simulink model "wind_turbine_2021"  (R2024a)
settings: Solver=VariableStepAuto  StartTime=0.0  StopTime=20.0  RelTol=1e-3
values from neighbouring files (symbols this model uses):
  a1 = 0.4    [parameter_definition.m]
  a2 = 0.25    [parameter_definition.m]
  Cp_coef = coeffvalues(surf_fit)    [wind_turbine_sim.m]
  Ct_coef = coeffvalues(surf_fit)    [wind_turbine_sim.m]
  Kv = sqrt(2 * Tv * (1 - a2^2) / (a1^2/a2 - a2 + 1 - a1^2))    [parameter_definition.m]
  Noise_power = 1    [parameter_definition.m]
  Noise_Ts = 0.001    [parameter_definition.m]
  R = 125.88 / 2    (= 62.94)    [surface_fitting.m]
  Tv = Lm / Vm    (= 25)    [parameter_definition.m]
  Vm = 6    [parameter_definition.m]
undefined symbols (not defined in the file or in its folder): Nb, rho
libraries: simulink x1
settings Model: Creator=User  LastModifiedBy=ml4
settings OptimizationCC: ReuseModelBlockBuffer=off
settings RTWCC: GPUComputeCapability=3.5

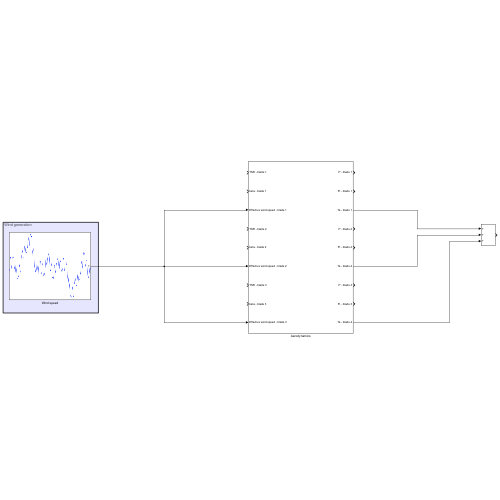
[thumbnail: Simulink's stored preview of the top-level diagram]
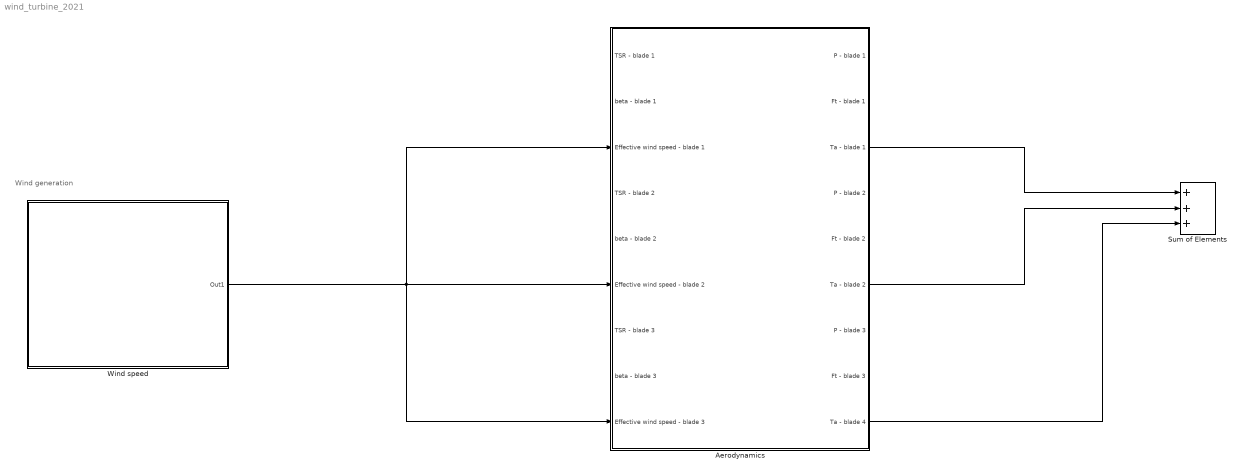
== system wind_turbine_2021 ==
  note: Wind generation
  Aerodynamics : Subsystem
  Sum of Elements : Sum  Inputs=+++
  Wind speed : Subsystem
      mask Display: image('./images/The-profile-of-the-wind-speed-versus-time.png');
  wires:
  Wind speed/1(Out1) -> Aerodynamics/3(Effective wind speed - blade 1), Aerodynamics/6(Effective wind speed - blade 2), Aerodynamics/9(Effective wind speed - blade 3)
  Aerodynamics/3(Ta - blade 1) -> Sum of Elements/1
  Aerodynamics/6(Ta - blade 2) -> Sum of Elements/2
  Aerodynamics/9(Ta - blade 4) -> Sum of Elements/3

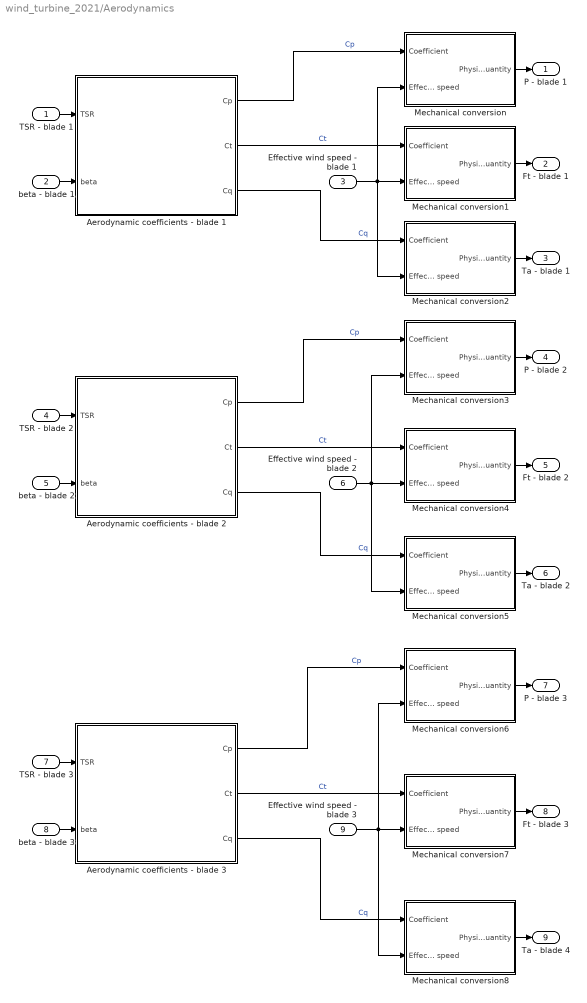
== system wind_turbine_2021/Aerodynamics ==
  TSR - blade 1 : Inport
  beta - blade 1 : Inport  Port=2
  Effective wind speed - blade 1 : Inport  Port=3
  TSR - blade 2 : Inport  Port=4
  beta - blade 2 : Inport  Port=5
  Effective wind speed - blade 2 : Inport  Port=6
  TSR - blade 3 : Inport  Port=7
  beta - blade 3 : Inport  Port=8
  Effective wind speed - blade 3 : Inport  Port=9
  Aerodynamic coefficients - blade 1 : Subsystem
      mask Display: image('C:\Users\User\Desktop\Project_repos\Controlab\Controlab\controlab\physical_models\2023\wind_turbine\images\Surface_fit.png'); % Use "Edit Image" on toolstrip to change.
  Aerodynamic coefficients - blade 2 : Subsystem
      mask Display: image('C:\Users\User\Desktop\Project_repos\Controlab\Controlab\controlab\physical_models\2023\wind_turbine\images\Surface_fit.png'); % Use "Edit Image" on toolstrip to change.
  Aerodynamic coefficients - blade 3 : Subsystem
      mask Display: image('C:\Users\User\Desktop\Project_repos\Controlab\Controlab\controlab\physical_models\2023\wind_turbine\images\Surface_fit.png'); % Use "Edit Image" on toolstrip to change.
  Mechanical conversion : Subsystem
  Mechanical conversion1 : Subsystem
  Mechanical conversion2 : Subsystem
  Mechanical conversion3 : Subsystem
  Mechanical conversion4 : Subsystem
  Mechanical conversion5 : Subsystem
  Mechanical conversion6 : Subsystem
  Mechanical conversion7 : Subsystem
  Mechanical conversion8 : Subsystem
  P - blade 1 : Outport
  Ft - blade 1 : Outport  Port=2
  Ta - blade 1 : Outport  Port=3
  P - blade 2 : Outport  Port=4
  Ft - blade 2 : Outport  Port=5
  Ta - blade 2 : Outport  Port=6
  P - blade 3 : Outport  Port=7
  Ft - blade 3 : Outport  Port=8
  Ta - blade 4 : Outport  Port=9
  wires:
  Aerodynamic coefficients - blade 1/1(Cp) -> Mechanical conversion/1(Coefficient)  "Cp"
  Aerodynamic coefficients - blade 3/3(Cq) -> Mechanical conversion8/1(Coefficient)  "Cq"
  Aerodynamic coefficients - blade 3/1(Cp) -> Mechanical conversion6/1(Coefficient)  "Cp"
  Aerodynamic coefficients - blade 3/2(Ct) -> Mechanical conversion7/1(Coefficient)  "Ct"
  beta - blade 1/1 -> Aerodynamic coefficients - blade 1/2(beta)
  Mechanical conversion5/1(Physical quantity) -> Ta - blade 2/1
  Aerodynamic coefficients - blade 2/3(Cq) -> Mechanical conversion5/1(Coefficient)  "Cq"
  Aerodynamic coefficients - blade 2/2(Ct) -> Mechanical conversion4/1(Coefficient)  "Ct"
  beta - blade 3/1 -> Aerodynamic coefficients - blade 3/2(beta)
  Aerodynamic coefficients - blade 2/1(Cp) -> Mechanical conversion3/1(Coefficient)  "Cp"
  Effective wind speed - blade 1/1 -> Mechanical conversion/2(Effective wind speed), Mechanical conversion1/2(Effective wind speed), Mechanical conversion2/2(Effective wind speed)
  Aerodynamic coefficients - blade 1/2(Ct) -> Mechanical conversion1/1(Coefficient)  "Ct"
  Aerodynamic coefficients - blade 1/3(Cq) -> Mechanical conversion2/1(Coefficient)  "Cq"
  TSR - blade 2/1 -> Aerodynamic coefficients - blade 2/1(TSR)
  Mechanical conversion6/1(Physical quantity) -> P - blade 3/1
  beta - blade 2/1 -> Aerodynamic coefficients - blade 2/2(beta)
  Mechanical conversion8/1(Physical quantity) -> Ta - blade 4/1
  Effective wind speed - blade 3/1 -> Mechanical conversion6/2(Effective wind speed), Mechanical conversion8/2(Effective wind speed), Mechanical conversion7/2(Effective wind speed)
  Mechanical conversion3/1(Physical quantity) -> P - blade 2/1
  TSR - blade 1/1 -> Aerodynamic coefficients - blade 1/1(TSR)
  TSR - blade 3/1 -> Aerodynamic coefficients - blade 3/1(TSR)
  Mechanical conversion/1(Physical quantity) -> P - blade 1/1
  Effective wind speed - blade 2/1 -> Mechanical conversion3/2(Effective wind speed), Mechanical conversion4/2(Effective wind speed), Mechanical conversion5/2(Effective wind speed)
  Mechanical conversion4/1(Physical quantity) -> Ft - blade 2/1
  Mechanical conversion1/1(Physical quantity) -> Ft - blade 1/1
  Mechanical conversion2/1(Physical quantity) -> Ta - blade 1/1
  Mechanical conversion7/1(Physical quantity) -> Ft - blade 3/1

== system wind_turbine_2021/Wind speed ==
  Band-Limited White Noise : simulink/Sources/Band-Limited White Noise  Cov=[Noise_power]  Ts=Noise_Ts  seed=[23341]
  Constant : Constant  Value=Vm
  Gain : Gain  Gain=Kv
  Sum of Elements : Sum
  Transfer Fcn : TransferFcn  Numerator=[Tv*a1 1]  Denominator=[(Tv^2)*a2 Tv*(1+a2) 1]
  Out1 : Outport
  wires:
  Band-Limited White Noise/1 -> Transfer Fcn/1
  Transfer Fcn/1 -> Gain/1
  Gain/1 -> Sum of Elements/2
  Constant/1 -> Sum of Elements/1
  Sum of Elements/1 -> Out1/1

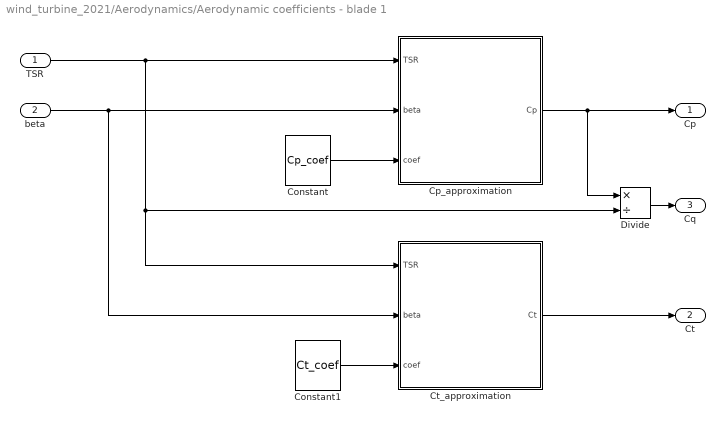
== system wind_turbine_2021/Aerodynamics/Aerodynamic coefficients - blade 1 ==
  TSR : Inport
  beta : Inport  Port=2
  Constant : Constant  Value=Cp_coef
  Constant1 : Constant  Value=Ct_coef
  Cp_approximation : MATLAB Function  TreatAsAtomicUnit=on
  Ct_approximation : MATLAB Function  TreatAsAtomicUnit=on
  Divide : Product  Inputs=*/
  Cp : Outport
  Ct : Outport  Port=2
  Cq : Outport  Port=3
  wires:
  Constant1/1 -> Ct_approximation/3(coef)
  Constant/1 -> Cp_approximation/3(coef)
  beta/1 -> Ct_approximation/2(beta), Cp_approximation/2(beta)
  Cp_approximation/1(Cp) -> Divide/1, Cp/1
  Ct_approximation/1(Ct) -> Ct/1
  TSR/1 -> Ct_approximation/1(TSR), Divide/2, Cp_approximation/1(TSR)
  Divide/1 -> Cq/1

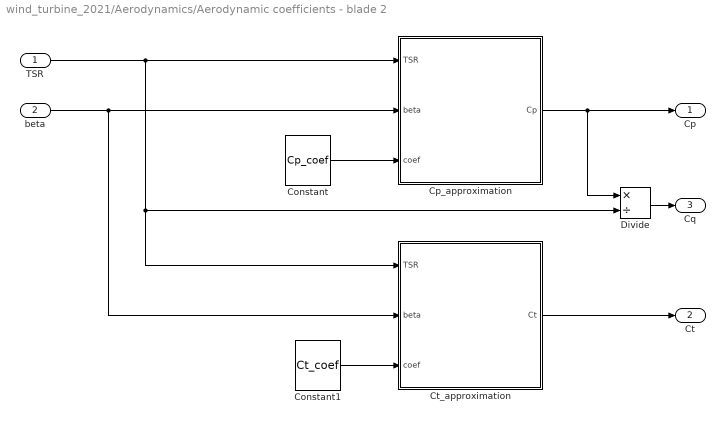
== system wind_turbine_2021/Aerodynamics/Aerodynamic coefficients - blade 2 ==
  TSR : Inport
  beta : Inport  Port=2
  Constant : Constant  Value=Cp_coef
  Constant1 : Constant  Value=Ct_coef
  Cp_approximation : MATLAB Function  TreatAsAtomicUnit=on
  Ct_approximation : MATLAB Function  TreatAsAtomicUnit=on
  Divide : Product  Inputs=*/
  Cp : Outport
  Ct : Outport  Port=2
  Cq : Outport  Port=3
  wires:
  Divide/1 -> Cq/1
  TSR/1 -> Cp_approximation/1(TSR), Divide/2, Ct_approximation/1(TSR)
  Ct_approximation/1(Ct) -> Ct/1
  Cp_approximation/1(Cp) -> Cp/1, Divide/1
  beta/1 -> Cp_approximation/2(beta), Ct_approximation/2(beta)
  Constant/1 -> Cp_approximation/3(coef)
  Constant1/1 -> Ct_approximation/3(coef)

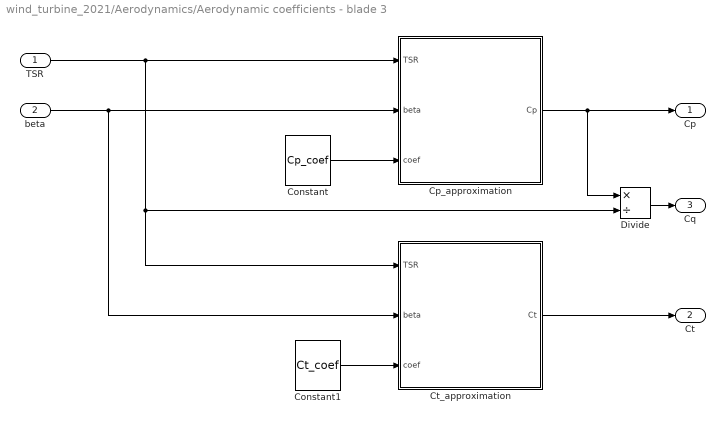
== system wind_turbine_2021/Aerodynamics/Aerodynamic coefficients - blade 3 ==
  TSR : Inport
  beta : Inport  Port=2
  Constant : Constant  Value=Cp_coef
  Constant1 : Constant  Value=Ct_coef
  Cp_approximation : MATLAB Function  TreatAsAtomicUnit=on
  Ct_approximation : MATLAB Function  TreatAsAtomicUnit=on
  Divide : Product  Inputs=*/
  Cp : Outport
  Ct : Outport  Port=2
  Cq : Outport  Port=3
  wires:
  Constant1/1 -> Ct_approximation/3(coef)
  Constant/1 -> Cp_approximation/3(coef)
  beta/1 -> Ct_approximation/2(beta), Cp_approximation/2(beta)
  Cp_approximation/1(Cp) -> Divide/1, Cp/1
  Ct_approximation/1(Ct) -> Ct/1
  TSR/1 -> Ct_approximation/1(TSR), Divide/2, Cp_approximation/1(TSR)
  Divide/1 -> Cq/1

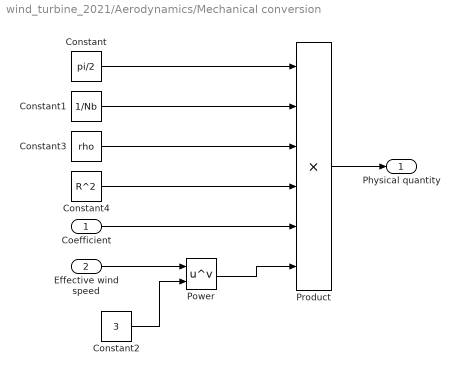
== system wind_turbine_2021/Aerodynamics/Mechanical conversion ==
  Coefficient : Inport
  Effective wind speed : Inport  Port=2
  Constant : Constant  Value=pi/2
  Constant1 : Constant  Value=1/Nb
  Constant2 : Constant  Value=3
  Constant3 : Constant  Value=rho
  Constant4 : Constant  Value=R^2
  Power : Math  Operator=pow
  Product : Product  Inputs=6
  Physical quantity : Outport
  wires:
  Coefficient/1 -> Product/5
  Constant1/1 -> Product/2
  Constant4/1 -> Product/4
  Constant/1 -> Product/1
  Product/1 -> Physical quantity/1
  Constant3/1 -> Product/3
  Effective wind speed/1 -> Power/1
  Power/1 -> Product/6
  Constant2/1 -> Power/2

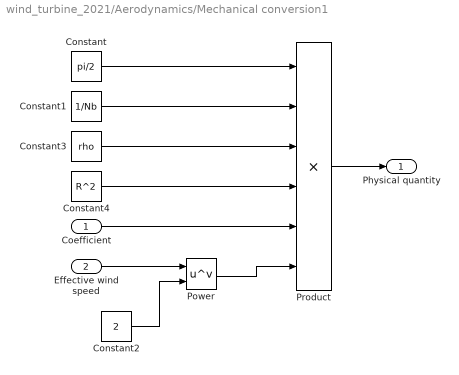
== system wind_turbine_2021/Aerodynamics/Mechanical conversion1 ==
  Coefficient : Inport
  Effective wind speed : Inport  Port=2
  Constant : Constant  Value=pi/2
  Constant1 : Constant  Value=1/Nb
  Constant2 : Constant  Value=2
  Constant3 : Constant  Value=rho
  Constant4 : Constant  Value=R^2
  Power : Math  Operator=pow
  Product : Product  Inputs=6
  Physical quantity : Outport
  wires:
  Constant3/1 -> Product/3
  Product/1 -> Physical quantity/1
  Constant/1 -> Product/1
  Constant4/1 -> Product/4
  Constant1/1 -> Product/2
  Coefficient/1 -> Product/5
  Constant2/1 -> Power/2
  Power/1 -> Product/6
  Effective wind speed/1 -> Power/1

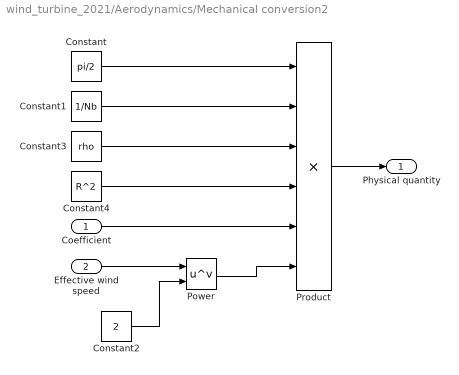
== system wind_turbine_2021/Aerodynamics/Mechanical conversion2 ==
  Coefficient : Inport
  Effective wind speed : Inport  Port=2
  Constant : Constant  Value=pi/2
  Constant1 : Constant  Value=1/Nb
  Constant2 : Constant  Value=2
  Constant3 : Constant  Value=rho
  Constant4 : Constant  Value=R^2
  Power : Math  Operator=pow
  Product : Product  Inputs=6
  Physical quantity : Outport
  wires:
  Coefficient/1 -> Product/5
  Constant1/1 -> Product/2
  Constant4/1 -> Product/4
  Constant/1 -> Product/1
  Product/1 -> Physical quantity/1
  Constant3/1 -> Product/3
  Power/1 -> Product/6
  Constant2/1 -> Power/2
  Effective wind speed/1 -> Power/1

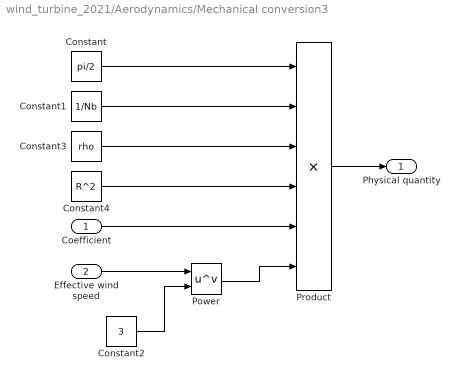
== system wind_turbine_2021/Aerodynamics/Mechanical conversion3 ==
  Coefficient : Inport
  Effective wind speed : Inport  Port=2
  Constant : Constant  Value=pi/2
  Constant1 : Constant  Value=1/Nb
  Constant2 : Constant  Value=3
  Constant3 : Constant  Value=rho
  Constant4 : Constant  Value=R^2
  Power : Math  Operator=pow
  Product : Product  Inputs=6
  Physical quantity : Outport
  wires:
  Constant3/1 -> Product/3
  Product/1 -> Physical quantity/1
  Constant/1 -> Product/1
  Constant4/1 -> Product/4
  Constant1/1 -> Product/2
  Coefficient/1 -> Product/5
  Effective wind speed/1 -> Power/1
  Constant2/1 -> Power/2
  Power/1 -> Product/6

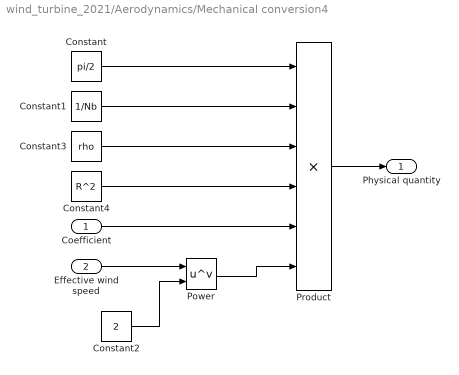
== system wind_turbine_2021/Aerodynamics/Mechanical conversion4 ==
  Coefficient : Inport
  Effective wind speed : Inport  Port=2
  Constant : Constant  Value=pi/2
  Constant1 : Constant  Value=1/Nb
  Constant2 : Constant  Value=2
  Constant3 : Constant  Value=rho
  Constant4 : Constant  Value=R^2
  Power : Math  Operator=pow
  Product : Product  Inputs=6
  Physical quantity : Outport
  wires:
  Coefficient/1 -> Product/5
  Constant1/1 -> Product/2
  Constant4/1 -> Product/4
  Constant/1 -> Product/1
  Product/1 -> Physical quantity/1
  Constant3/1 -> Product/3
  Power/1 -> Product/6
  Constant2/1 -> Power/2
  Effective wind speed/1 -> Power/1

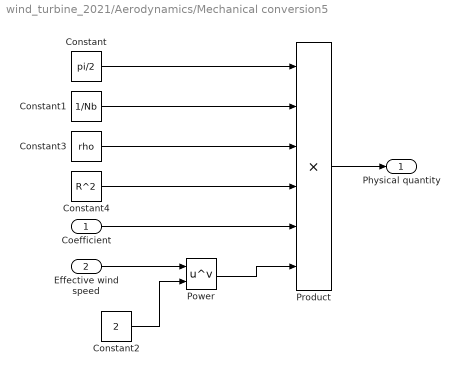
== system wind_turbine_2021/Aerodynamics/Mechanical conversion5 ==
  Coefficient : Inport
  Effective wind speed : Inport  Port=2
  Constant : Constant  Value=pi/2
  Constant1 : Constant  Value=1/Nb
  Constant2 : Constant  Value=2
  Constant3 : Constant  Value=rho
  Constant4 : Constant  Value=R^2
  Power : Math  Operator=pow
  Product : Product  Inputs=6
  Physical quantity : Outport
  wires:
  Constant3/1 -> Product/3
  Product/1 -> Physical quantity/1
  Constant/1 -> Product/1
  Constant4/1 -> Product/4
  Constant1/1 -> Product/2
  Coefficient/1 -> Product/5
  Power/1 -> Product/6
  Constant2/1 -> Power/2
  Effective wind speed/1 -> Power/1

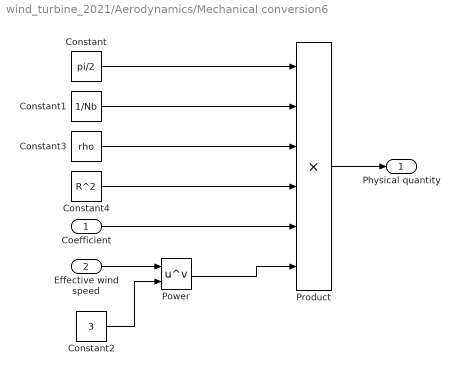
== system wind_turbine_2021/Aerodynamics/Mechanical conversion6 ==
  Coefficient : Inport
  Effective wind speed : Inport  Port=2
  Constant : Constant  Value=pi/2
  Constant1 : Constant  Value=1/Nb
  Constant2 : Constant  Value=3
  Constant3 : Constant  Value=rho
  Constant4 : Constant  Value=R^2
  Power : Math  Operator=pow
  Product : Product  Inputs=6
  Physical quantity : Outport
  wires:
  Coefficient/1 -> Product/5
  Constant1/1 -> Product/2
  Constant4/1 -> Product/4
  Constant/1 -> Product/1
  Product/1 -> Physical quantity/1
  Constant3/1 -> Product/3
  Constant2/1 -> Power/2
  Power/1 -> Product/6
  Effective wind speed/1 -> Power/1

== system wind_turbine_2021/Aerodynamics/Mechanical conversion7 ==
  Coefficient : Inport
  Effective wind speed : Inport  Port=2
  Constant : Constant  Value=pi/2
  Constant1 : Constant  Value=1/Nb
  Constant2 : Constant  Value=2
  Constant3 : Constant  Value=rho
  Constant4 : Constant  Value=R^2
  Power : Math  Operator=pow
  Product : Product  Inputs=6
  Physical quantity : Outport
  wires:
  Constant3/1 -> Product/3
  Product/1 -> Physical quantity/1
  Constant/1 -> Product/1
  Constant4/1 -> Product/4
  Constant1/1 -> Product/2
  Coefficient/1 -> Product/5
  Power/1 -> Product/6
  Constant2/1 -> Power/2
  Effective wind speed/1 -> Power/1

== system wind_turbine_2021/Aerodynamics/Mechanical conversion8 ==
  Coefficient : Inport
  Effective wind speed : Inport  Port=2
  Constant : Constant  Value=pi/2
  Constant1 : Constant  Value=1/Nb
  Constant2 : Constant  Value=2
  Constant3 : Constant  Value=rho
  Constant4 : Constant  Value=R^2
  Power : Math  Operator=pow
  Product : Product  Inputs=6
  Physical quantity : Outport
  wires:
  Coefficient/1 -> Product/5
  Constant1/1 -> Product/2
  Constant4/1 -> Product/4
  Constant/1 -> Product/1
  Product/1 -> Physical quantity/1
  Constant3/1 -> Product/3
  Power/1 -> Product/6
  Constant2/1 -> Power/2
  Effective wind speed/1 -> Power/1

== matlab function wind_turbine_2021/Aerodynamics/Aerodynamic coefficients - blade 1/Cp_approximation ==
  data: TSR input; Cp output; beta input; coef input
function Cp = Cp_fitting(TSR, beta, coef)

Cp = coef(1) + coef(2) * TSR + coef(3) * beta + ...
     coef(4) * TSR^2 + coef(5) * TSR * beta + coef(6) * beta^2 + ...
     coef(7) * TSR^3 + coef(8) * TSR^2 * beta + coef(9) * TSR * beta^2 + coef(10) * beta^3 + ...
     coef(11) * TSR^4 + coef(12) * TSR^3 * beta + coef(13) * TSR^2 * beta^2 + coef(14) * TSR * beta^3 + coef(15) * beta^4 + ...
     coef(16) * TSR^5 + coef(17) * TSR^4 * beta + coef(18) * TSR^3 * beta^2 + coef(19) * TSR^2 * beta^3 + coef(20) * TSR * beta^4 + coef(21) * beta^5;

== matlab function wind_turbine_2021/Aerodynamics/Aerodynamic coefficients - blade 2/Cp_approximation ==
  data: TSR input; Cp output; beta input; coef input
function Cp = Cp_fitting(TSR, beta, coef)

Cp = coef(1) + coef(2) * TSR + coef(3) * beta + ...
     coef(4) * TSR^2 + coef(5) * TSR * beta + coef(6) * beta^2 + ...
     coef(7) * TSR^3 + coef(8) * TSR^2 * beta + coef(9) * TSR * beta^2 + coef(10) * beta^3 + ...
     coef(11) * TSR^4 + coef(12) * TSR^3 * beta + coef(13) * TSR^2 * beta^2 + coef(14) * TSR * beta^3 + coef(15) * beta^4 + ...
     coef(16) * TSR^5 + coef(17) * TSR^4 * beta + coef(18) * TSR^3 * beta^2 + coef(19) * TSR^2 * beta^3 + coef(20) * TSR * beta^4 + coef(21) * beta^5;

== matlab function wind_turbine_2021/Aerodynamics/Aerodynamic coefficients - blade 2/Ct_approximation ==
  data: TSR input; Ct output; beta input; coef input
function Ct = Ct_fitting(TSR, beta, coef)

Ct = coef(1) + coef(2) * TSR + coef(3) * beta + ...
     coef(4) * TSR^2 + coef(5) * TSR * beta + coef(6) * beta^2 + ...
     coef(7) * TSR^3 + coef(8) * TSR^2 * beta + coef(9) * TSR * beta^2 + coef(10) * beta^3 + ...
     coef(11) * TSR^4 + coef(12) * TSR^3 * beta + coef(13) * TSR^2 * beta^2 + coef(14) * TSR * beta^3 + coef(15) * beta^4 + ...
     coef(16) * TSR^5 + coef(17) * TSR^4 * beta + coef(18) * TSR^3 * beta^2 + coef(19) * TSR^2 * beta^3 + coef(20) * TSR * beta^4 + coef(21) * beta^5;

== matlab function wind_turbine_2021/Aerodynamics/Aerodynamic coefficients - blade 3/Cp_approximation ==
  data: TSR input; Cp output; beta input; coef input
function Cp = Cp_fitting(TSR, beta, coef)

Cp = coef(1) + coef(2) * TSR + coef(3) * beta + ...
     coef(4) * TSR^2 + coef(5) * TSR * beta + coef(6) * beta^2 + ...
     coef(7) * TSR^3 + coef(8) * TSR^2 * beta + coef(9) * TSR * beta^2 + coef(10) * beta^3 + ...
     coef(11) * TSR^4 + coef(12) * TSR^3 * beta + coef(13) * TSR^2 * beta^2 + coef(14) * TSR * beta^3 + coef(15) * beta^4 + ...
     coef(16) * TSR^5 + coef(17) * TSR^4 * beta + coef(18) * TSR^3 * beta^2 + coef(19) * TSR^2 * beta^3 + coef(20) * TSR * beta^4 + coef(21) * beta^5;

== matlab function wind_turbine_2021/Aerodynamics/Aerodynamic coefficients - blade 3/Ct_approximation ==
  data: TSR input; Ct output; beta input; coef input
function Ct = Ct_fitting(TSR, beta, coef)

Ct = coef(1) + coef(2) * TSR + coef(3) * beta + ...
     coef(4) * TSR^2 + coef(5) * TSR * beta + coef(6) * beta^2 + ...
     coef(7) * TSR^3 + coef(8) * TSR^2 * beta + coef(9) * TSR * beta^2 + coef(10) * beta^3 + ...
     coef(11) * TSR^4 + coef(12) * TSR^3 * beta + coef(13) * TSR^2 * beta^2 + coef(14) * TSR * beta^3 + coef(15) * beta^4 + ...
     coef(16) * TSR^5 + coef(17) * TSR^4 * beta + coef(18) * TSR^3 * beta^2 + coef(19) * TSR^2 * beta^3 + coef(20) * TSR * beta^4 + coef(21) * beta^5;

== matlab function wind_turbine_2021/Aerodynamics/Aerodynamic coefficients - blade 1/Ct_approximation ==
  data: TSR input; Ct output; beta input; coef input
function Ct = Ct_fitting(TSR, beta, coef)

Ct = coef(1) + coef(2) * TSR + coef(3) * beta + ...
     coef(4) * TSR^2 + coef(5) * TSR * beta + coef(6) * beta^2 + ...
     coef(7) * TSR^3 + coef(8) * TSR^2 * beta + coef(9) * TSR * beta^2 + coef(10) * beta^3 + ...
     coef(11) * TSR^4 + coef(12) * TSR^3 * beta + coef(13) * TSR^2 * beta^2 + coef(14) * TSR * beta^3 + coef(15) * beta^4 + ...
     coef(16) * TSR^5 + coef(17) * TSR^4 * beta + coef(18) * TSR^3 * beta^2 + coef(19) * TSR^2 * beta^3 + coef(20) * TSR * beta^4 + coef(21) * beta^5;
